simulink model "Lab_6"  (R2014a)
settings: Solver=ode23t  StartTime=0.0  StopTime=20  RelTol=1e-3
undefined symbols (not defined in the file or in its folder): DZ, SL
libraries: simulink x1
settings Model: Creator=cloughj  LastModifiedBy=cloughj
settings SolverCC: ZeroCrossAlgorithm=Adaptive

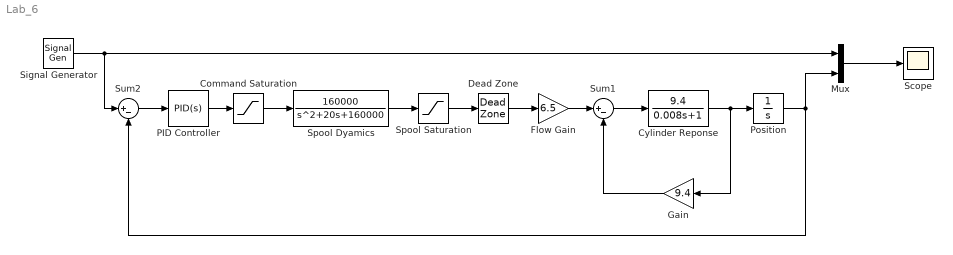
== system Lab_6 ==
  Command Saturation : Saturate  UpperLimit=SL  LowerLimit=-SL
  Cylinder Reponse : TransferFcn  Numerator=[9.4]  Denominator="[0.008  1]"
  Dead Zone : DeadZone  LowerValue=-DZ  UpperValue=DZ  SaturateOnIntegerOverflow=on
  Flow Gain : Gain  Gain=6.5
  Gain : Gain  Gain=9.4
  Mux : Mux  Inputs=2
  PID Controller : simulink/Continuous/PID Controller  Controller=PID  TimeDomain=Continuous-time  SampleTime=1  IntegratorMethod=Forward Euler  FilterMethod=Forward Euler  Form=Parallel  P=100  I=0.1  D=0  N=100  InitialConditionSource=internal  InitialConditionForIntegrator=0  InitialConditionForFilter=0  ExternalReset=none  LimitOutput=off  UpperSaturationLimit=inf  LowerSaturationLimit=-inf  LinearizeAsGain=on  AntiWindupMode=none  Kb=1  TrackingMode=off  Kt=1  PParamMin=[]  PParamMax=[]  IParamMin=[]  IParamMax=[]  DParamMin=[]  DParamMax=[]  NParamMin=[]  NParamMax=[]  KbParamMin=[]  KbParamMax=[]  KtParamMin=[]  KtParamMax=[]  POutMin=[]  POutMax=[]  IOutMin=[]  IOutMax=[]  DOutMin=[]  DOutMax=[]  NOutMin=[]  NOutMax=[]  KbOutMin=[]  KbOutMax=[]  KtOutMin=[]  KtOutMax=[]  IntegratorOutMin=[]  IntegratorOutMax=[]  FilterOutMin=[]  FilterOutMax=[]  SumOutMin=[]  SumOutMax=[]  SumI1OutMin=[]  SumI1OutMax=[]  SumI2OutMin=[]  SumI2OutMax=[]  SumI3OutMin=[]  SumI3OutMax=[]  SumDOutMin=[]  SumDOutMax=[]  SaturationOutMin=[]  SaturationOutMax=[]  IntegratorContinuousStateAttributes=''  IntegratorStateMustResolveToSignalObject=off  IntegratorRTWStateStorageClass=Auto  FilterContinuousStateAttributes=''  FilterStateMustResolveToSignalObject=off  FilterRTWStateStorageClass=Auto
  Position : Integrator
  Scope : Scope
  Signal Generator : SignalGenerator  WaveForm=square  Amplitude=3  Frequency=0.1
  Spool Saturation : Saturate  UpperLimit=SL  LowerLimit=-SL
  Spool Dyamics : TransferFcn  Numerator=[160000]  Denominator=[1 20 160000]
  Sum1 : Sum  Inputs=|+-
  Sum2 : Sum  Inputs=|+-
  wires:
  Mux/1 -> Scope/1
  Signal Generator/1 -> Sum2/1, Mux/1
  Sum2/1 -> PID Controller/1
  PID Controller/1 -> Command Saturation/1
  Command Saturation/1 -> Spool Dyamics/1
  Spool Dyamics/1 -> Spool Saturation/1
  Spool Saturation/1 -> Dead Zone/1
  Dead Zone/1 -> Flow Gain/1
  Flow Gain/1 -> Sum1/1
  Sum1/1 -> Cylinder Reponse/1
  Cylinder Reponse/1 -> Gain/1, Position/1
  Gain/1 -> Sum1/2
  Position/1 -> Sum2/2, Mux/2
